simulink model "Capacitor Braking_Indhu Kanth"  (R2013a)
settings: Solver=ode45  StartTime=0.0  StopTime=10  RelTol=1e-3
libraries: powerlib x14, powerlib_extras x3, simulink x2
settings Model: Creator=Indhu Kanth  LastModifiedBy=Indhu Kanth

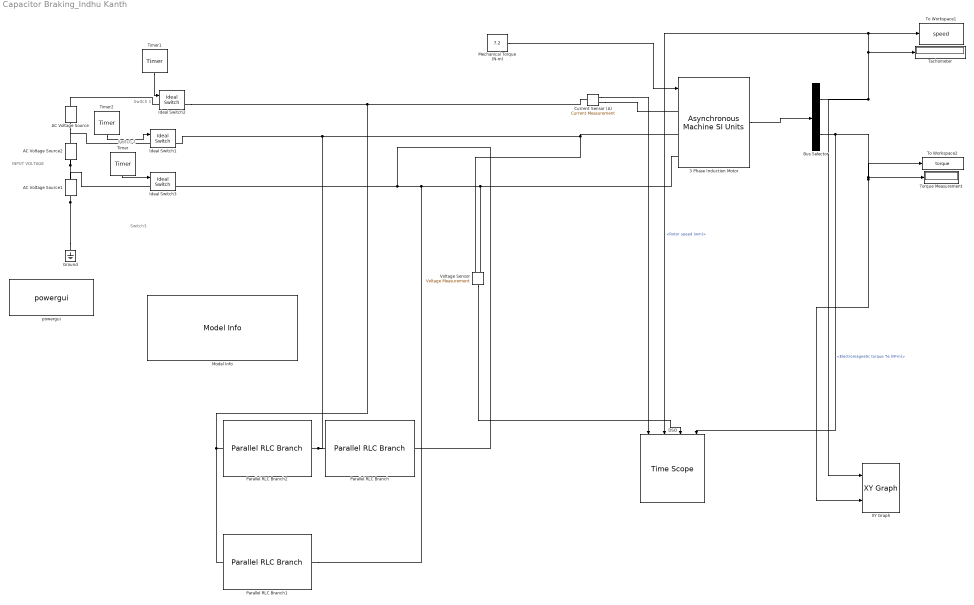
== system Capacitor Braking_Indhu Kanth ==
  note: INPUT VOLTAGE
  note: Switch3
  note: Switch 2
  note: Switch 1
  3 Phase Induction Motor : powerlib/Machines/Asynchronous Machine SI Units  PresetModel=No  MechanicalLoad=Torque Tm  ShowDetailedParameters=on  RotorType=Squirrel-cage  ReferenceFrame=Rotor  NominalParameters=[2200 415 50]  Stator=[1.405 0.005839]  Rotor=[1.395 0.005839]  Cage1=[ 0.022 0.226/377]  Cage2=[ 0.022 0.226/377]  Lm=0.1722  Mechanical=[0.0131 0.002985 2]  PolePairs=2  InitialConditions=[1 0 0 0 0 0 0 0]  Units=SI  LoadFlowParameters=1492000  SimulateSaturation=off  Saturation=[14.03593122, 27.81365428, 53.79336849, 72.68890987, 97.98006896, 148.6815601, 215.7428561, 302.9841135, 428.7778367 ; 230, 322, 414, 460, 506, 552, 598, 644, 690]  TsPowergui=0  TsBlock=-1  IterativeModel=Forward Euler  Pmec=0
  AC Voltage Source : powerlib/Electrical Sources/AC Voltage Source  Amplitude=200*sqrt(2)  Phase=0  Frequency=50  SampleTime=0  Measurements=Voltage
  AC Voltage Source1 : powerlib/Electrical Sources/AC Voltage Source  Amplitude=200*sqrt(2)  Phase=120  Frequency=50  SampleTime=0  Measurements=Voltage
  AC Voltage Source2 : powerlib/Electrical Sources/AC Voltage Source  Amplitude=200*sqrt(2)  Phase=-120  Frequency=50  SampleTime=0  Measurements=Voltage
  Bus Selector : BusSelector  OutputSignals=Mechanical.Rotor speed (wm),Mechanical.Electromagnetic torque Te (N*m)
  Current Sensor (A) : powerlib/Measurements/Current Measurement  PhasorSimulation=off  OutputType=Complex  PSBequivalent=0
  DSO : TimeScope  NumInputPorts=4  DefaultConfigurationName=spbscopes.TimeScopeBlockCfg
      settings: CopyFcn=scopeextensions.ScopeBlock.callback(gcbh, 'onBlockCopy', gcbh);  DeleteFcn=scopeextensions.ScopeBlock.callback(gcbh, 'onBlockDelete');  PreSaveFcn=scopeextensions.ScopeBlock.callback(gcbh, 'onModelSave');  NameChangeFcn=scopeextensions.ScopeBlock.callback(gcbh, 'onBlockRename');  CloseFcn=scopeextensions.ScopeBlock.callback(gcbh, 'onBlockClose');  PreDeleteFcn=scopeextensions.ScopeBlock.callback(gcbh, 'onBlockPreDelete');
  Ground : powerlib/Elements/Ground  LConnTagsString=a
  Ideal Switch1 : powerlib/Power Electronics/Ideal Switch  Ron=0.001  Lon=0  IC=1  Rs=1e5  Cs=inf  Measurements=on
  Ideal Switch2 : powerlib/Power Electronics/Ideal Switch  Ron=0.001  Lon=0  IC=1  Rs=1e5  Cs=inf  Measurements=on
  Ideal Switch3 : powerlib/Power Electronics/Ideal Switch  Ron=0.001  Lon=0  IC=1  Rs=1e5  Cs=inf  Measurements=on
  Mechanical Torque (N-m) : Constant  Value=7.2
  Model Info : simulink/Model-Wide Utilities/Model Info  InitialBlockCM=None  BlockCM=None  Frame=on  DisplayStringWithTags=|  HorizontalTextAlignment=Center  LeftAlignmentValue=0.5  SourceBlockDiagram=selfstudycapacitorbraking  TagMaxNumber=20
      | 3 PHASE INDUCTION MOTOR
      | Capacitor Braking
      | Indhy Kanth
  Parallel RLC Branch : powerlib/Elements/Parallel RLC Branch  LConnTagsString=a  RConnTagsString=__new0  BranchType=C  Resistance=1  Inductance=1e-3  SetiL0=off  InitialCurrent=0  Capacitance=100  Setx0=off  InitialVoltage=0  Measurements=None
  Parallel RLC Branch1 : powerlib/Elements/Parallel RLC Branch  LConnTagsString=a  RConnTagsString=__new0  BranchType=C  Resistance=1  Inductance=1e-3  SetiL0=off  InitialCurrent=0  Capacitance=100  Setx0=off  InitialVoltage=0  Measurements=None
  Parallel RLC Branch2 : powerlib/Elements/Parallel RLC Branch  LConnTagsString=a  RConnTagsString=__new0  BranchType=C  Resistance=1  Inductance=1e-3  SetiL0=off  InitialCurrent=0  Capacitance=100  Setx0=off  InitialVoltage=0  Measurements=None
  Tachometer : Display
  Timer : powerlib_extras/Control  Blocks/Timer  t=[0 5 ]  e="[1  0 ]"
  Timer1 : powerlib_extras/Control  Blocks/Timer  t="[0  5 ]"  e="[1  0 ]"
  Timer2 : powerlib_extras/Control  Blocks/Timer  t=[0 5 ]  e="[1  0 ]"
  To Workspace1 : ToWorkspace  VariableName=speed  SampleTime=-1
  To Workspace2 : ToWorkspace  VariableName=torque  SampleTime=-1
  Torque Measurement : Display
  Voltage Sensor : powerlib/Measurements/Voltage Measurement  PhasorSimulation=off  OutputType=Complex  PSBequivalent=0
  XY Graph : simulink/Sinks/XY Graph  xmin=-0.2  xmax=0.2  ymin=-0.1  ymax=0.1  st=-1
  powergui : powerlib/powergui  Priority=1  SimulationMode=Continuous  SolverType=Tustin  SampleTime=50e-6  frequency=60  SPID=off  DisableSnubberDevices=off  DisableRonSwitches=off  DisableVfSwitches=off  SwTol=0  Interpol=off  DisplayEquations=off  frequencyindice=50  Pbase=100e6  ErrMax=1e-4  Iterations=50  UnitsV=kV  UnitsW=MW  FunctionMessages=off  echomessages=off  HookPort=off  EnableUseOfTLC=off  x0status=blocks  RestoreLinks=warning  ResistiveCurrentMeasurement=off  Frange=[0:2:500]  Ylog=off  Xlog=on  ShowGrid=off  save=off  variable=ZData  ZoomFFT=on  StartTime=0.0  cycles=1  DisplayStyle=1  fundamental=60  FreqAxis=off  MaxFrequency=1000  frequencyindicesteady=1  RmsSteady=1  display=off  Ts=0  methode=off
  wires:
  Mechanical Torque (N-m)/1 -> 3 Phase Induction Motor/1
  Timer1/1 -> Ideal Switch2/1
  Timer2/1 -> Ideal Switch1/1
  Timer/1 -> Ideal Switch3/1
  3 Phase Induction Motor/1 -> Bus Selector/1
  Current Sensor (A)/1 -> DSO/1
  Bus Selector/1 -> XY Graph/1, DSO/2, To Workspace1/1, Tachometer/1  "<Rotor speed (wm)>"
  Bus Selector/2 -> To Workspace2/1, Torque Measurement/1, XY Graph/2, DSO/4  "<Electromagnetic torque Te (N*m)>"
  Voltage Sensor/1 -> DSO/3
  connections:
  Ground/LConn1 -- AC Voltage Source1/LConn1 -- AC Voltage Source/LConn1 -- AC Voltage Source2/LConn1
  Ideal Switch2/RConn1 -- Parallel RLC Branch1/LConn1 -- Parallel RLC Branch2/LConn1 -- Current Sensor (A)/LConn1
  Voltage Sensor/LConn1 -- 3 Phase Induction Motor/LConn2 -- Parallel RLC Branch/LConn1 -- Parallel RLC Branch2/RConn1 -- Ideal Switch1/RConn1
  Voltage Sensor/LConn2 -- 3 Phase Induction Motor/LConn3 -- Parallel RLC Branch1/RConn1 -- Parallel RLC Branch/RConn1 -- Ideal Switch3/RConn1
  Ideal Switch2/LConn1 -- AC Voltage Source/RConn1
  Ideal Switch1/LConn1 -- AC Voltage Source2/RConn1
  AC Voltage Source1/RConn1 -- Ideal Switch3/LConn1
  Current Sensor (A)/RConn1 -- 3 Phase Induction Motor/LConn1
